simulink model "rlwatertank"  (R2022b)
settings: Solver=FixedStepAuto  StartTime=0.0  StopTime=200.0  FixedStep=0.1  RelTol=1e-3  EnableMultiTasking=on
settings Model: DataDictionary=BusSystem.sldd  Creator=The MathWorks, Inc.  LastModifiedBy=Robert
settings SolverCC: AlgebraicLoopSolver=TrustRegion
settings DataIOCC: LimitDataPoints=on  SaveOutput=off  ReturnWorkspaceOutputs=off  SignalLoggingName=logsOut
settings OptimizationCC: ExpressionDepthLimit=2147483647  InitFltsAndDblsToZero=on  LifeSpan=inf
settings DebuggingCC: SaveWithParameterizedLinksMsg=none  UnderspecifiedInitializationDetection=Classic  MergeDetectMultiDrivingBlocksExec=none  SignalResolutionControl=TryResolveAllWithWarning  MultiTaskDSMMsg=warning  FcnCallInpInsideContextMsg=warning  UnconnectedInputMsg=warning  UnconnectedOutputMsg=warning  UnconnectedLineMsg=warning  AllowSymbolicDim=off  StateNameClashWarn=warning  SFUnexpectedBacktrackingDiag=warning  SFNoUnconditionalDefaultTransitionDiag=warning  SFExecutionAtInitializationDiag=none  SFMachineParentedDataDiag=warning  ArithmeticOperatorsInVariantConditions=warning
settings HardwareCC: ProdBitPerPointer=32  ProdBitPerSizeT=32  ProdBitPerPtrDiffT=32  ProdLargestAtomicFloat=None  ProdIntDivRoundTo=Undefined  ProdEndianess=Unspecified  ProdWordSize=32  ProdHWDeviceType=Specified
settings ModelReferenceCC: EnableRefExpFcnMdlSchedulingChecks=on  PropagateSignalLabelsOutOfModel=off
settings SFSimCC: SimUseLocalCustomCode=off  CustomCodeUndefinedFunction=UseInterfaceOnly
settings RTWCC: RTWUseLocalCustomCode=off  DLArmComputeVersion=19.05
settings CodeAppCC: StateflowObjectComments=on
settings GRTTargetCC: TargetFcnLib=ansi_tfl_tmw.mat  TargetLangStandard=C89/C90 (ANSI)  CombineOutputUpdateFcns=off  GRTInterface=on
settings ConfigComp: CovMetricSettings=dw  CovSaveCumulativeToWorkspaceVar=on  CovSaveSingleToWorkspaceVar=on  CovExternalEMLEnable=off

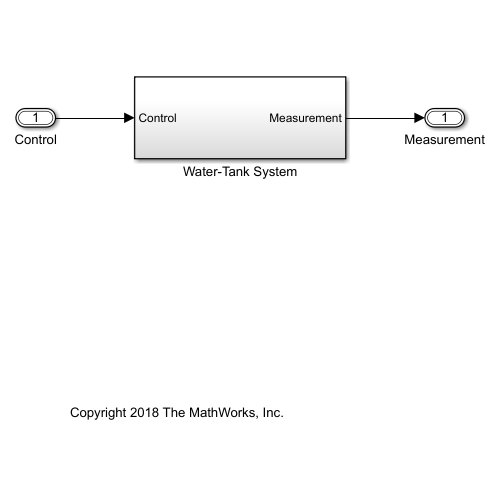
[thumbnail: Simulink's stored preview of the top-level diagram]
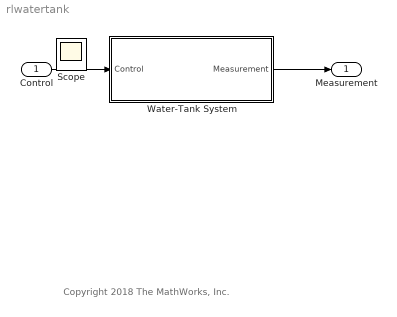
== system rlwatertank ==
  note: Copyright 2018 The MathWorks, Inc.
  Control : Inport  OutDataTypeStr=Bus: Control
  Water-Tank System : Subsystem
  Measurement : Outport  OutDataTypeStr=Bus: slBus2
  Scope : Scope
  wires:
  Control/1 -> Water-Tank System/1(Control)
  Water-Tank System/1(Measurement) -> Measurement/1

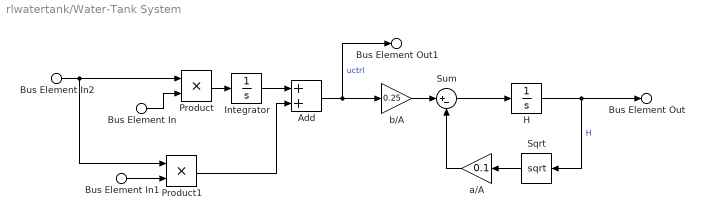
== system rlwatertank/Water-Tank System ==
  Bus Element In2 : Inport  PortName=Control  Element=Error
  Bus Element In : Inport  PortName=Control  Element=KI
  Bus Element In1 : Inport  PortName=Control  Element=KP
  Add : Sum
  H : Integrator  InitialCondition=3  LimitOutput=on  LowerSaturationLimit=0
  Integrator : Integrator
  Product : Product
  Product1 : Product
  Sqrt : Sqrt  OutputSignalType=real
  Sum : Sum  Inputs=|+-  SaturateOnIntegerOverflow=on
  a/A : Gain  Gain=0.1  SaturateOnIntegerOverflow=on  OutDataTypeStr=Inherit: Same as input  ParamDataTypeStr=Inherit: Same as input
  b/A : Gain  Gain=0.25  SaturateOnIntegerOverflow=on  OutDataTypeStr=Inherit: Same as input  ParamDataTypeStr=Inherit: Same as input
  Bus Element Out : Outport  PortName=Measurement  Element=Height
  Bus Element Out1 : Outport  PortName=Measurement  Element=uctrl
  wires:
  Bus Element In2/1 -> Product1/1, Product/1
  Bus Element In/1 -> Product/2
  Product1/1 -> Add/2
  Bus Element In1/1 -> Product1/2
  Product/1 -> Integrator/1
  Sum/1 -> H/1
  Integrator/1 -> Add/1
  a/A/1 -> Sum/2
  b/A/1 -> Sum/1
  Add/1 -> Bus Element Out1/1, b/A/1  "uctrl"
  H/1 -> Bus Element Out/1, Sqrt/1  "H"
  Sqrt/1 -> a/A/1
